simulink subsystem "IdealVoltageSource"  (R2022b)
settings: Solver=VariableStepAuto  StartTime=0.0  StopTime=10.0  RelTol=1e-3
undefined symbols (not defined in the file): PlntBattIdealSoc, PlntBattIdealVolt
settings Model: ModifiedByFormat=The MathWorks, Inc.  Creator=The MathWorks, Inc.  LastModifiedBy=The MathWorks, Inc.
settings SolverCC: MaxZcPerStep=1
settings DebuggingCC: UnconnectedInputMsg=warning  UnconnectedOutputMsg=warning  UnconnectedLineMsg=warning
settings ModelReferenceCC: EnableRefExpFcnMdlSchedulingChecks=on
settings RTWCC: DLArmComputeVersion=19.05

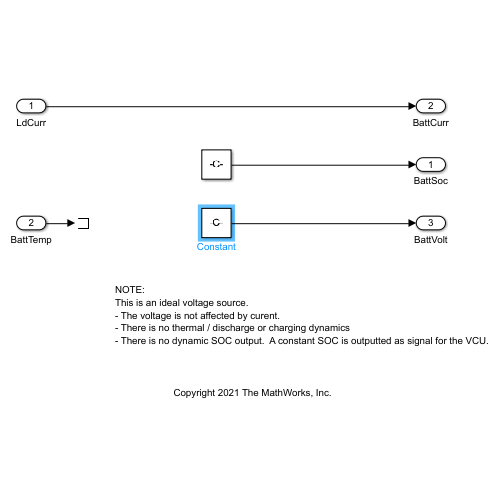
[thumbnail: Simulink's stored preview of the top-level diagram]
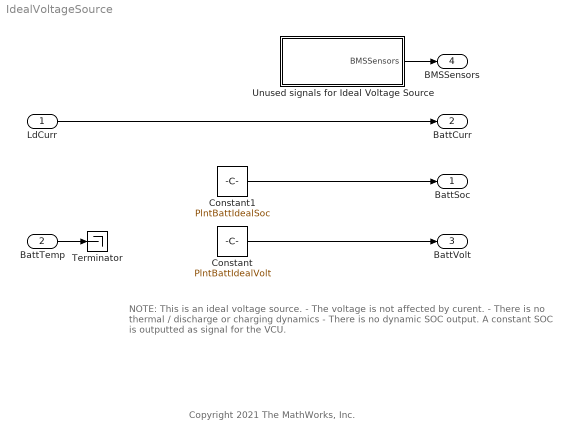
== system IdealVoltageSource ==
  note: Copyright 2021 The MathWorks, Inc.
  note: NOTE:
      | This is an ideal voltage source.
      | - The voltage is not affected by curent.
      | - There is no thermal / discharge or charging dynamics
      | - There is no dynamic SOC output.  A constant SOC is outputted as signal for the VCU.
  LdCurr : Inport
  BattTemp : Inport  Port=2
  Constant : Constant  Value=PlntBattIdealVolt  SampleTime=-1
  Constant1 : Constant  Value=PlntBattIdealSoc  SampleTime=-1
  Terminator : Terminator
  Unused signals for Ideal Voltage Source : Subsystem
  BattSoc : Outport  VectorParamsAs1DForOutWhenUnconnected=off
  BattCurr : Outport  Port=2  VectorParamsAs1DForOutWhenUnconnected=off
  BattVolt : Outport  Port=3  VectorParamsAs1DForOutWhenUnconnected=off
  BMSSensors : Outport  Port=4  VectorParamsAs1DForOutWhenUnconnected=off
  wires:
  Constant/1 -> BattVolt/1
  BattTemp/1 -> Terminator/1
  LdCurr/1 -> BattCurr/1
  Constant1/1 -> BattSoc/1
  Unused signals for Ideal Voltage Source/1(BMSSensors) -> BMSSensors/1

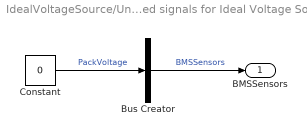
== system IdealVoltageSource/Unused signals for Ideal Voltage Source ==
  Bus Creator : BusCreator  Inputs=1
  Constant : Constant  Value=0  SampleTime=-1
  BMSSensors : Outport
  wires:
  Bus Creator/1 -> BMSSensors/1  "BMSSensors"
  Constant/1 -> Bus Creator/1  "PackVoltage"
